simulink model "CCModel_71"  (R2024a)
settings: Solver=ode3  StartTime=0.0  StopTime=100  FixedStep=0.001  RelTol=1e-3  EnableMultiTasking=on
undefined symbols (not defined in the file or in its folder): DiscIntNeverNeededParam, Hecate_desVel1, Hecate_desVel2, Hecate_desVel3, Hecate_horShift, Hecate_period, Hecate_slope, Hecate_Transition1, Hecate_Transition2, Hecate_verShift, i, PME_qb, qb_map, RPM_qb, V
libraries: simulink x46
(part 6 of 11)

== system CCModel_71/Cruise Control/Version 7.3/PID Controller ==
  Error : Inport
  Source : Inport  Port=2
  Desired Velocity : Inport  Port=3
  Add : Sum
  Derivative : Derivative
  Gain : Gain  Gain=0.17
  Integrator : Integrator  ExternalReset=rising
  Kd : Gain  Gain=0.1
  Ki : Gain  Gain=0.0075
  Kp : Gain  Gain=4.2
  Polynomial : Polyval  Coefs=[0.0000428571, -0.0079428571, 0.5357142857, 0]
  Sum : Sum  Inputs=+++
  Switch : Switch  Criteria=u2 > Threshold  Threshold=100  SaturateOnIntegerOverflow=off  InputSameDT=off
  Throttle Adjustment : Subsystem
  u : Outport
  wires:
  Integrator/1 -> Ki/1
  Error/1 -> Kp/1, Derivative/1, Integrator/1
  Derivative/1 -> Kd/1
  Source/1 -> Integrator/2  "Integral reset"
  Desired Velocity/1 -> Polynomial/1, Switch/2, Gain/1
  Sum/1 -> Add/1
  Add/1 -> u/1
  Switch/1 -> Add/2
  Gain/1 -> Switch/3
  Polynomial/1 -> Switch/1
  Kd/1 -> Sum/1  "D"
  Kp/1 -> Sum/2  "P"
  Ki/1 -> Sum/3  "I"

== system CCModel_71/Cruise Control/Version 7.3/Sigmoid ==
  U1 : Inport
  U2 : Inport  Port=2
  Change_time : Inport  Port=3
  Abs : Abs  SaturateOnIntegerOverflow=off
  Abs2 : Abs  SaturateOnIntegerOverflow=off
  Add Constant : Bias  Bias=1  SaturateOnIntegerOverflow=off
  Add Constant2 : Bias  Bias=1  SaturateOnIntegerOverflow=off
  Add Constant3 : Bias  Bias=1  SaturateOnIntegerOverflow=off
  Add3 : Sum
  Add4 : Sum  Inputs=+-
  Add5 : Sum
  Clock1 : Clock
  Constant : Constant
  Constant3 : Constant
  Divide : Product  Inputs=/*
  Divide1 : Product  Inputs=**
  Divide4 : Product  Inputs=*/
  Divide5 : Product  Inputs=**
  Divide6 : Product  Inputs=**
  Divide8 : Product  Inputs=*/
  Gain : Gain  Gain=1/2
  Gain1 : Gain  Gain=2
  Gain2 : Gain  Gain=1000
  Gain3 : Gain  Gain=0.001
  Gain5 : Gain  Gain=1/2
  K : Constant  Value=4
  Power{,3..5} (4 alike) : Math  Operator=pow
  Reciprocal : Product  Inputs=/
  Reciprocal2 : Product  Inputs=/
  Round1 : Rounding  Operator=round
  Saturation : Saturate  UpperLimit=100  LowerLimit=-100
  Subtract : Sum  Inputs=+-
  Subtract1 : Sum  Inputs=+-
  Subtract2 : Sum  Inputs=+-
  Sum1 : Sum  Inputs=|-+
  h : Constant
  u_out : Outport
  wires:
  Add5/1 -> Saturation/1
  h/1 -> Divide8/1, Abs2/1, Subtract/2
  Add3/1 -> Divide6/2
  Add4/1 -> Divide5/1
  Constant3/1 -> Add4/1, Add3/2
  Power5/1 -> Divide4/2
  Reciprocal2/1 -> Power5/2
  K/1 -> Reciprocal2/1, Power4/2, Power/2, Reciprocal/1
  Gain5/1 -> Divide6/1
  Change_time/1 -> Sum1/1
  Abs/1 -> Power4/1
  Clock1/1 -> Sum1/2
  Gain3/1 -> Subtract/1
  U2/1 -> Gain5/1, Divide1/2
  Round1/1 -> Gain3/1
  Power4/1 -> Add Constant/1
  Gain2/1 -> Round1/1
  Add Constant/1 -> Power5/1
  Subtract/1 -> Divide4/1, Abs/1
  U1/1 -> Subtract2/1
  Divide6/1 -> Add5/1
  Sum1/1 -> Gain2/1
  Divide4/1 -> Add3/1, Add4/2
  Abs2/1 -> Power/1
  Power/1 -> Add Constant2/1
  Add Constant2/1 -> Power3/1
  Reciprocal/1 -> Power3/2
  Power3/1 -> Divide8/2
  Divide8/1 -> Add Constant3/1
  Add Constant3/1 -> Gain/1
  Constant/1 -> Subtract1/1
  Gain/1 -> Gain1/1, Subtract1/2  "P"
  Divide1/1 -> Subtract2/2
  Subtract2/1 -> Divide/2
  Gain1/1 -> Divide/1
  Divide/1 -> Divide5/2
  Divide5/1 -> Add5/2
  Saturation/1 -> u_out/1
  Subtract1/1 -> Divide1/1

== system CCModel_71/Cruise Control/Version 7.3/Switches ==
  U : Inport
  Throttle_In : Inport  Port=2
  Brake_In : Inport  Port=3
  Add Constant : Bias  Bias=6  SaturateOnIntegerOverflow=off
  Brake_Switch1 : Switch  Criteria=u2 > Threshold  Threshold=30  SaturateOnIntegerOverflow=off  InputSameDT=off
  Brake_Switch3 : Switch  Criteria=u2 > Threshold  Threshold=5  SaturateOnIntegerOverflow=off  InputSameDT=off
  Constant1 : Constant  Value=0
  Gain : Gain  Gain=-1
  Gain3 : Gain  Gain=0.15
  Max1 : MinMax  Function=max  Inputs=2
  Polynomial : Polyval  Coefs=[-0.01,0.2,0,0]
  Polynomial1 : Polyval  Coefs=[6.66666666666666666666666666666666666e-7,-9.33333333333333333333333333333333e-05,0.0105,-0.448,6]
  Saturation : Saturate  UpperLimit=100  LowerLimit=-100
  Switch : Switch  Criteria=u2 > Threshold  Threshold=10  SaturateOnIntegerOverflow=off  InputSameDT=off
  Switch1 : Switch  Criteria=u2 > Threshold  Threshold=-20  SaturateOnIntegerOverflow=off  InputSameDT=off
  Throttle_Switch1 : Switch  Criteria=u2 > Threshold  SaturateOnIntegerOverflow=off  InputSameDT=off
  Throttle_Switch3 : Switch  Criteria=u2 > Threshold  Threshold=5  SaturateOnIntegerOverflow=off  InputSameDT=off
  To Workspace : ToWorkspace  VariableName=throttleout  SampleTime=-1
      settings: Save2DSignal=2-D array (concatenate along first dimension)
  To Workspace1 : ToWorkspace  VariableName=brakeout  SampleTime=-1
      settings: Save2DSignal=2-D array (concatenate along first dimension)
  Throttle : Outport
  Brake : Outport  Port=2
  wires:
  Throttle_Switch1/1 -> Add Constant/1
  Brake_Switch3/1 -> To Workspace1/1, Brake/1
  Brake_In/1 -> Brake_Switch3/1, Max1/2
  Throttle_In/1 -> Throttle_Switch3/1, Max1/1
  Throttle_Switch3/1 -> Saturation/1
  Constant1/1 -> Throttle_Switch1/3, Brake_Switch1/1
  Switch/1 -> Throttle_Switch1/1
  Polynomial/1 -> Switch/3
  Max1/1 -> Brake_Switch3/2, Throttle_Switch3/2
  Add Constant/1 -> Throttle_Switch3/3
  Gain/1 -> Switch1/3
  Polynomial1/1 -> Switch1/1
  Switch1/1 -> Brake_Switch1/3
  Brake_Switch1/1 -> Gain3/1
  Gain3/1 -> Brake_Switch3/3
  Saturation/1 -> To Workspace/1, Throttle/1
  U/1 -> Switch1/2, Brake_Switch1/2, Throttle_Switch1/2, Gain/1, Switch/2, Switch/1, Polynomial/1, Polynomial1/1

== system CCModel_71/Powertrain/EM0/efficiency ==
  Motor speed [rpm] : Inport
  "Torque [Nm] " : Inport  Port=2
  Abs : Abs  SaturateOnIntegerOverflow=off
  Abs2 : Abs  SaturateOnIntegerOverflow=off
  Inverter efficiency : Gain  Gain=0.97
  Inverter efficiency1 : Gain  Gain=0.97
  Multiply : Gain  Gain=1/9.5488
  Product{,1..2,5} (4 alike) : Product
  Product3 : Product  Inputs=3
  Product4 : Product  Inputs=3
  RPM to rad/s : Gain  Gain=0.104719755
  RPM to rad/s1 : Gain  Gain=0.104719755
  Saturation : Saturate  UpperLimit=inf  LowerLimit=0
  Saturation1 : Saturate  UpperLimit=0  LowerLimit=-inf
  Saturation2 : Saturate  UpperLimit=inf  LowerLimit=0
  Saturation3 : Saturate  UpperLimit=inf  LowerLimit=0
  Sign : Signum  ZeroCross=off
  Subtract : Sum  Inputs=+-
  Subtract1 : Sum  Inputs=+-
  Switch : Switch  Criteria=u2 > Threshold  ZeroCross=off  SaturateOnIntegerOverflow=off  InputSameDT=off
  Terminator : Terminator
  Terminator1 : Terminator
  divider : Subsystem
  divider1 : Subsystem
  motor efficiency map : Lookup_n-D  BreakpointsForDimension1=|  BreakpointsForDimension2="[1\t440.500000000000\t881\t1321.50000000000\t1762\t2202.50000000000\t2643\t3083.50000000000\t3524\t3964.50000000000\t4405\t4845.50000000000\t5286\t5726.50000000000\t6167\t6607.50000000000\t7048\t7488.50000000000\t7929\t8369.50000000000\t8810]"  Table=|  InternalRulePriority=Speed  RndMeth=Simplest
      BreakpointsForDimension1=|
      | [1
      | 6
      | 12
      | 18
      | 36
      | 54
      | 72
      | 90
      | 108
      | 126
      | 144
      | 162
      | 180
      | 198
      | 216
      | 234
      | 252
      | 270
      | 288
      | 306
      | 324
      | 342
      | 360]
      Table=|
      | [0.100000000000000	0.100000000000000	0.420000000000000	0.440000000000000	0.450000000000000	0.460000000000000	0.470000000000000	0.480000000000000	0.490000000000000	0.500000000000000	0.510000000000000	0.520000000000000	0.530000000000000	0.540000000000000	0.550000000000000	0.560000000000000	0.580000000000000	0.560000000000000	0.550000000000000	0.540000000000000	0.500000000000000
      | 0.740000000000000	0.750000000000000	0.750000000000000	0.760000000000000	0.763000000000000	0.767000000000000	0.780000000000000	0.780000000000000	0.780000000000000	0.780000000000000	0.780000000000000	0.770000000000000	0.770000000000000	0.770000000000000	0.769000000000000	0.769000000000000	0.765000000000000	0.760000000000000	0.750000000000000	0.730000000000000	0.720000000000000
      | 0.780000000000000	0.790000000000000	0.800000000000000	0.850000000000000	0.880000000000000	0.890000000000000	0.895000000000000	0.900000000000000	0.910000000000000	0.910000000000000	0.910000000000000	0.915000000000000	0.915000000000000	0.918000000000000	0.917000000000000	0.916000000000000	0.910000000000000	0.910000000000000	0.894000000000000	0.870000000000000	0.850000000000000
      | 0.800000000000000	0.870000000000000	0.902500000000000	0.942500000000000	0.945000000000000	0.945000000000000	0.945000000000000	0.945000000000000	0.945000000000000	0.947500000000000	0.945000000000000	0.945000000000000	0.945000000000000	0.945000000000000	0.945000000000000	0.937500000000000	0.920000000000000	0.910000000000000	0.898000000000000	0.890000000000000	0.840000000000000
      | 0.800000000000000	0.880000000000000	0.902500000000000	0.947500000000000	0.953000000000000	0.955000000000000	0.957500000000000	0.957500000000000	0.956000000000000	0.960000000000000	0.960000000000000	0.960000000000000	0.960000000000000	0.957500000000000	0.957500000000000	0.955000000000000	0.950000000000000	0.945000000000000	0.940000000000000	0.920000000000000	0.890000000000000
      | 0.780000000000000	0.880000000000000	0.902500000000000	0.947500000000000	0.952500000000000	0.957500000000000	0.960000000000000	0.962000000000000	0.962500000000000	0.964000000000000	0.965000000000000	0.965000000000000	0.965000000000000	0.965000000000000	0.962500000000000	0.958000000000000	0.957000000000000	0.951000000000000	0.947500000000000	0.945000000000000	0.940000000000000
      | 0.740000000000000	0.880000000000000	0.902500000000000	0.942500000000000	0.952500000000000	0.955000000000000	0.962000000000000	0.964000000000000	0.966000000000000	0.967000000000000	0.968000000000000	0.970000000000000	0.967000000000000	0.966000000000000	0.964000000000000	0.962000000000000	0.960000000000000	0.956000000000000	0.953000000000000	0.948000000000000	0.945000000000000
      | 0.700000000000000	0.870000000000000	0.902500000000000	0.945000000000000	0.947500000000000	0.952500000000000	0.960000000000000	0.962500000000000	0.965000000000000	0.966000000000000	0.968000000000000	0.970000000000000	0.967500000000000	0.966500000000000	0.965000000000000	0.962500000000000	0.960000000000000	0.955000000000000	0.952000000000000	0.946000000000000	0.945000000000000
      | 0.650000000000000	0.860000000000000	0.902500000000000	0.932500000000000	0.942500000000000	0.950000000000000	0.957500000000000	0.961000000000000	0.963000000000000	0.965500000000000	0.967500000000000	0.970000000000000	0.967500000000000	0.965000000000000	0.964000000000000	0.960000000000000	0.957000000000000	0.953000000000000	0.950000000000000	0.945000000000000	0.942000000000000
      | 0.600000000000000	0.850000000000000	0.902500000000000	0.927500000000000	0.937500000000000	0.947500000000000	0.955000000000000	0.959000000000000	0.962500000000000	0.965000000000000	0.966000000000000	0.967500000000000	0.965000000000000	0.963000000000000	0.961800000000000	0.957500000000000	0.955000000000000	0.950000000000000	0.945000000000000	0.941000000000000	0.937500000000000
      | 0.590000000000000	0.840000000000000	0.902500000000000	0.925000000000000	0.932500000000000	0.942500000000000	0.952500000000000	0.957500000000000	0.960000000000000	0.962500000000000	0.965000000000000	0.965000000000000	0.962500000000000	0.961000000000000	0.958000000000000	0.954000000000000	0.950000000000000	0.945000000000000	0.940000000000000	0.930000000000000	0.925000000000000
      | 0.550000000000000	0.830000000000000	0.902500000000000	0.922500000000000	0.927500000000000	0.937500000000000	0.950000000000000	0.955000000000000	0.957500000000000	0.961000000000000	0.962500000000000	0.962500000000000	0.960000000000000	0.957500000000000	0.955000000000000	0.950000000000000	0.945000000000000	0.935000000000000	0.922500000000000	0.917500000000000	0.915000000000000
      | 0.540000000000000	0.820000000000000	0.890000000000000	0.920000000000000	0.922500000000000	0.935000000000000	0.947000000000000	0.952000000000000	0.955000000000000	0.958000000000000	0.961200000000000	0.960000000000000	0.957500000000000	0.954000000000000	0.950000000000000	0.942500000000000	0.932500000000000	0.922500000000000	0.912500000000000	0.910000000000000	0
      | 0.500000000000000	0.810000000000000	0.880000000000000	0.910000000000000	0.920000000000000	0.930000000000000	0.942500000000000	0.951250000000000	0.952500000000000	0.956000000000000	0.960000000000000	0.956000000000000	0.952500000000000	0.950000000000000	0.942500000000000	0.930000000000000	0.915000000000000	0.910000000000000	0	0	0
      | 0.450000000000000	0.805000000000000	0.870000000000000	0.905000000000000	0.917500000000000	0.925000000000000	0.940000000000000	0.945000000000000	0.950000000000000	0.952500000000000	0.955000000000000	0.952500000000000	0.948000000000000	0.942500000000000	0.930000000000000	0.915000000000000	0.910000000000000	0	0	0	0
      | 0.430000000000000	0.800000000000000	0.860000000000000	0.890000000000000	0.912500000000000	0.920000000000000	0.935000000000000	0.942500000000000	0.946000000000000	0.950000000000000	0.952500000000000	0.949000000000000	0.942500000000000	0.935000000000000	0.917500000000000	0.912500000000000	0	0	0	0	0
      | 0.420000000000000	0.790000000000000	0.850000000000000	0.880000000000000	0.907500000000000	0.915000000000000	0.932000000000000	0.937500000000000	0.942500000000000	0.945000000000000	0.948000000000000	0.942500000000000	0.935000000000000	0.922500000000000	0.915000000000000	0	0	0	0	0	0
      | 0.410000000000000	0.780000000000000	0.840000000000000	0.870000000000000	0.900000000000000	0.910000000000000	0.927500000000000	0.935000000000000	0.938000000000000	0.942500000000000	0.945000000000000	0.935000000000000	0.925000000000000	0.920000000000000	0	0	0	0	0	0	0
      | 0.400000000000000	0.760000000000000	0.830000000000000	0.860000000000000	0.890000000000000	0.905000000000000	0.922500000000000	0.930000000000000	0.935000000000000	0.937500000000000	0.935000000000000	0.927500000000000	0	0	0	0	0	0	0	0	0
      | 0.380000000000000	0.740000000000000	0.820000000000000	0.850000000000000	0.880000000000000	0.900000000000000	0.917500000000000	0.927500000000000	0.930000000000000	0.930000000000000	0.922500000000000	0.920000000000000	0	0	0	0	0	0	0	0	0
      | 0.360000000000000	0.710000000000000	0.810000000000000	0.840000000000000	0.875000000000000	0.897500000000000	0.912500000000000	0.922500000000000	0.925000000000000	0.928000000000000	0.915000000000000	0	0	0	0	0	0	0	0	0	0
      | 0.350000000000000	0.700000000000000	0.800000000000000	0.835000000000000	0.872500000000000	0.880000000000000	0.905000000000000	0.917500000000000	0.921000000000000	0.920000000000000	0	0	0	0	0	0	0	0	0	0	0
      | 0.350000000000000	0.680000000000000	0.790000000000000	0.830000000000000	0.870000000000000	0.875000000000000	0.900000000000000	0.910000000000000	0.900000000000000	0	0	0	0	0	0	0	0	0	0	0	0]
      settings: InputPortMap=u0,u1
  motor efficiency map1 : Lookup_n-D  BreakpointsForDimension1=|  BreakpointsForDimension2="[1\t440.500000000000\t881\t1321.50000000000\t1762\t2202.50000000000\t2643\t3083.50000000000\t3524\t3964.50000000000\t4405\t4845.50000000000\t5286\t5726.50000000000\t6167\t6607.50000000000\t7048\t7488.50000000000\t7929\t8369.50000000000\t8810]"  Table=|  InternalRulePriority=Speed  RndMeth=Simplest
      BreakpointsForDimension1=|
      | [1
      | 6
      | 12
      | 18
      | 36
      | 54
      | 72
      | 90
      | 108
      | 126
      | 144
      | 162
      | 180
      | 198
      | 216
      | 234
      | 252
      | 270
      | 288
      | 306
      | 324
      | 342
      | 360]
      Table=|
      | [0.100000000000000	0.100000000000000	0.420000000000000	0.440000000000000	0.450000000000000	0.460000000000000	0.470000000000000	0.480000000000000	0.490000000000000	0.500000000000000	0.510000000000000	0.520000000000000	0.530000000000000	0.540000000000000	0.550000000000000	0.560000000000000	0.580000000000000	0.560000000000000	0.550000000000000	0.540000000000000	0.500000000000000
      | 0.740000000000000	0.750000000000000	0.750000000000000	0.760000000000000	0.763000000000000	0.767000000000000	0.780000000000000	0.780000000000000	0.780000000000000	0.780000000000000	0.780000000000000	0.770000000000000	0.770000000000000	0.770000000000000	0.769000000000000	0.769000000000000	0.765000000000000	0.760000000000000	0.750000000000000	0.730000000000000	0.720000000000000
      | 0.780000000000000	0.790000000000000	0.800000000000000	0.850000000000000	0.880000000000000	0.890000000000000	0.895000000000000	0.900000000000000	0.910000000000000	0.910000000000000	0.910000000000000	0.915000000000000	0.915000000000000	0.918000000000000	0.917000000000000	0.916000000000000	0.910000000000000	0.910000000000000	0.894000000000000	0.870000000000000	0.850000000000000
      | 0.800000000000000	0.870000000000000	0.902500000000000	0.942500000000000	0.945000000000000	0.945000000000000	0.945000000000000	0.945000000000000	0.945000000000000	0.947500000000000	0.945000000000000	0.945000000000000	0.945000000000000	0.945000000000000	0.945000000000000	0.937500000000000	0.920000000000000	0.910000000000000	0.898000000000000	0.890000000000000	0.840000000000000
      | 0.800000000000000	0.880000000000000	0.902500000000000	0.947500000000000	0.953000000000000	0.955000000000000	0.957500000000000	0.957500000000000	0.956000000000000	0.960000000000000	0.960000000000000	0.960000000000000	0.960000000000000	0.957500000000000	0.957500000000000	0.955000000000000	0.950000000000000	0.945000000000000	0.940000000000000	0.920000000000000	0.890000000000000
      | 0.780000000000000	0.880000000000000	0.902500000000000	0.947500000000000	0.952500000000000	0.957500000000000	0.960000000000000	0.962000000000000	0.962500000000000	0.964000000000000	0.965000000000000	0.965000000000000	0.965000000000000	0.965000000000000	0.962500000000000	0.958000000000000	0.957000000000000	0.951000000000000	0.947500000000000	0.945000000000000	0.940000000000000
      | 0.740000000000000	0.880000000000000	0.902500000000000	0.942500000000000	0.952500000000000	0.955000000000000	0.962000000000000	0.964000000000000	0.966000000000000	0.967000000000000	0.968000000000000	0.970000000000000	0.967000000000000	0.966000000000000	0.964000000000000	0.962000000000000	0.960000000000000	0.956000000000000	0.953000000000000	0.948000000000000	0.945000000000000
      | 0.700000000000000	0.870000000000000	0.902500000000000	0.945000000000000	0.947500000000000	0.952500000000000	0.960000000000000	0.962500000000000	0.965000000000000	0.966000000000000	0.968000000000000	0.970000000000000	0.967500000000000	0.966500000000000	0.965000000000000	0.962500000000000	0.960000000000000	0.955000000000000	0.952000000000000	0.946000000000000	0.945000000000000
      | 0.650000000000000	0.860000000000000	0.902500000000000	0.932500000000000	0.942500000000000	0.950000000000000	0.957500000000000	0.961000000000000	0.963000000000000	0.965500000000000	0.967500000000000	0.970000000000000	0.967500000000000	0.965000000000000	0.964000000000000	0.960000000000000	0.957000000000000	0.953000000000000	0.950000000000000	0.945000000000000	0.942000000000000
      | 0.600000000000000	0.850000000000000	0.902500000000000	0.927500000000000	0.937500000000000	0.947500000000000	0.955000000000000	0.959000000000000	0.962500000000000	0.965000000000000	0.966000000000000	0.967500000000000	0.965000000000000	0.963000000000000	0.961800000000000	0.957500000000000	0.955000000000000	0.950000000000000	0.945000000000000	0.941000000000000	0.937500000000000
      | 0.590000000000000	0.840000000000000	0.902500000000000	0.925000000000000	0.932500000000000	0.942500000000000	0.952500000000000	0.957500000000000	0.960000000000000	0.962500000000000	0.965000000000000	0.965000000000000	0.962500000000000	0.961000000000000	0.958000000000000	0.954000000000000	0.950000000000000	0.945000000000000	0.940000000000000	0.930000000000000	0.925000000000000
      | 0.550000000000000	0.830000000000000	0.902500000000000	0.922500000000000	0.927500000000000	0.937500000000000	0.950000000000000	0.955000000000000	0.957500000000000	0.961000000000000	0.962500000000000	0.962500000000000	0.960000000000000	0.957500000000000	0.955000000000000	0.950000000000000	0.945000000000000	0.935000000000000	0.922500000000000	0.917500000000000	0.915000000000000
      | 0.540000000000000	0.820000000000000	0.890000000000000	0.920000000000000	0.922500000000000	0.935000000000000	0.947000000000000	0.952000000000000	0.955000000000000	0.958000000000000	0.961200000000000	0.960000000000000	0.957500000000000	0.954000000000000	0.950000000000000	0.942500000000000	0.932500000000000	0.922500000000000	0.912500000000000	0.910000000000000	0
      | 0.500000000000000	0.810000000000000	0.880000000000000	0.910000000000000	0.920000000000000	0.930000000000000	0.942500000000000	0.951250000000000	0.952500000000000	0.956000000000000	0.960000000000000	0.956000000000000	0.952500000000000	0.950000000000000	0.942500000000000	0.930000000000000	0.915000000000000	0.910000000000000	0	0	0
      | 0.450000000000000	0.805000000000000	0.870000000000000	0.905000000000000	0.917500000000000	0.925000000000000	0.940000000000000	0.945000000000000	0.950000000000000	0.952500000000000	0.955000000000000	0.952500000000000	0.948000000000000	0.942500000000000	0.930000000000000	0.915000000000000	0.910000000000000	0	0	0	0
      | 0.430000000000000	0.800000000000000	0.860000000000000	0.890000000000000	0.912500000000000	0.920000000000000	0.935000000000000	0.942500000000000	0.946000000000000	0.950000000000000	0.952500000000000	0.949000000000000	0.942500000000000	0.935000000000000	0.917500000000000	0.912500000000000	0	0	0	0	0
      | 0.420000000000000	0.790000000000000	0.850000000000000	0.880000000000000	0.907500000000000	0.915000000000000	0.932000000000000	0.937500000000000	0.942500000000000	0.945000000000000	0.948000000000000	0.942500000000000	0.935000000000000	0.922500000000000	0.915000000000000	0	0	0	0	0	0
      | 0.410000000000000	0.780000000000000	0.840000000000000	0.870000000000000	0.900000000000000	0.910000000000000	0.927500000000000	0.935000000000000	0.938000000000000	0.942500000000000	0.945000000000000	0.935000000000000	0.925000000000000	0.920000000000000	0	0	0	0	0	0	0
      | 0.400000000000000	0.760000000000000	0.830000000000000	0.860000000000000	0.890000000000000	0.905000000000000	0.922500000000000	0.930000000000000	0.935000000000000	0.937500000000000	0.935000000000000	0.927500000000000	0	0	0	0	0	0	0	0	0
      | 0.380000000000000	0.740000000000000	0.820000000000000	0.850000000000000	0.880000000000000	0.900000000000000	0.917500000000000	0.927500000000000	0.930000000000000	0.930000000000000	0.922500000000000	0.920000000000000	0	0	0	0	0	0	0	0	0
      | 0.360000000000000	0.710000000000000	0.810000000000000	0.840000000000000	0.875000000000000	0.897500000000000	0.912500000000000	0.922500000000000	0.925000000000000	0.928000000000000	0.915000000000000	0	0	0	0	0	0	0	0	0	0
      | 0.350000000000000	0.700000000000000	0.800000000000000	0.835000000000000	0.872500000000000	0.880000000000000	0.905000000000000	0.917500000000000	0.921000000000000	0.920000000000000	0	0	0	0	0	0	0	0	0	0	0
      | 0.350000000000000	0.680000000000000	0.790000000000000	0.830000000000000	0.870000000000000	0.875000000000000	0.900000000000000	0.910000000000000	0.900000000000000	0	0	0	0	0	0	0	0	0	0	0	0]
      settings: InputPortMap=u0,u1
  Electrical power [W] : Outport
  wires:
  Switch/1 -> Electrical power [W]/1  "Elec_power"
  Sign/1 -> Switch/2
  Product1/1 -> Switch/3
  divider/1(Out1) -> Switch/1
  "Torque [Nm] "/1 -> Abs/1, Product5/1, Product4/2, Abs2/1, Product3/1, Product2/2, Product/2
  Product/1 -> Multiply/1
  motor efficiency map/1 -> Saturation2/1
  motor efficiency map1/1 -> Saturation3/1
  Abs/1 -> motor efficiency map1/1
  Motor speed [rpm]/1 -> motor efficiency map1/2, RPM to rad/s1/1, Product/1, RPM to rad/s/1, motor efficiency map/2
  Saturation3/1 -> Inverter efficiency1/1
  Saturation2/1 -> Inverter efficiency/1
  Abs2/1 -> motor efficiency map/1
  RPM to rad/s/1 -> Product3/2, Product2/1
  Product3/1 -> Subtract/2
  Product2/1 -> Subtract/1
  Subtract/1 -> divider1/1(In1)
  divider1/1(Out1) -> Saturation/1  "propelling"
  RPM to rad/s1/1 -> Product5/2, Product4/3
  Product4/1 -> Subtract1/1
  Product5/1 -> Subtract1/2
  Subtract1/1 -> Saturation1/1  "ReGen"
  Multiply/1 -> Product1/1, Sign/1, divider/1(In1)  "Mech_power"
  Inverter efficiency/1 -> divider1/2(In2), Product3/3, divider/2(In2)
  Inverter efficiency1/1 -> Product4/1, Product1/2
  Saturation/1 -> Terminator/1
  Saturation1/1 -> Terminator1/1

== system CCModel_71/Powertrain/EM1/efficiency ==
  Motor speed [rpm] : Inport
  "Torque [Nm] " : Inport  Port=2
  Abs : Abs  SaturateOnIntegerOverflow=off
  Abs2 : Abs  SaturateOnIntegerOverflow=off
  Inverter efficiency : Gain  Gain=0.97
  Inverter efficiency1 : Gain  Gain=0.97
  Multiply : Gain  Gain=1/9.5488
  Product{,1..2,5} (4 alike) : Product
  Product3 : Product  Inputs=3
  Product4 : Product  Inputs=3
  RPM to rad/s : Gain  Gain=0.104719755
  RPM to rad/s1 : Gain  Gain=0.104719755
  Saturation : Saturate  UpperLimit=inf  LowerLimit=0
  Saturation1 : Saturate  UpperLimit=0  LowerLimit=-inf
  Saturation2 : Saturate  UpperLimit=inf  LowerLimit=0
  Saturation3 : Saturate  UpperLimit=inf  LowerLimit=0
  Sign : Signum  ZeroCross=off
  Subtract : Sum  Inputs=+-
  Subtract1 : Sum  Inputs=+-
  Switch : Switch  Criteria=u2 > Threshold  ZeroCross=off  SaturateOnIntegerOverflow=off  InputSameDT=off
  Terminator : Terminator
  Terminator1 : Terminator
  divider : Subsystem
  divider1 : Subsystem
  motor efficiency map : Lookup_n-D  BreakpointsForDimension1=|  BreakpointsForDimension2="[1\t440.500000000000\t881\t1321.50000000000\t1762\t2202.50000000000\t2643\t3083.50000000000\t3524\t3964.50000000000\t4405\t4845.50000000000\t5286\t5726.50000000000\t6167\t6607.50000000000\t7048\t7488.50000000000\t7929\t8369.50000000000\t8810]"  Table=|  InternalRulePriority=Speed  RndMeth=Simplest
      BreakpointsForDimension1=|
      | [1
      | 6
      | 12
      | 18
      | 36
      | 54
      | 72
      | 90
      | 108
      | 126
      | 144
      | 162
      | 180
      | 198
      | 216
      | 234
      | 252
      | 270
      | 288
      | 306
      | 324
      | 342
      | 360]
      Table=|
      | [0.100000000000000	0.100000000000000	0.420000000000000	0.440000000000000	0.450000000000000	0.460000000000000	0.470000000000000	0.480000000000000	0.490000000000000	0.500000000000000	0.510000000000000	0.520000000000000	0.530000000000000	0.540000000000000	0.550000000000000	0.560000000000000	0.580000000000000	0.560000000000000	0.550000000000000	0.540000000000000	0.500000000000000
      | 0.740000000000000	0.750000000000000	0.750000000000000	0.760000000000000	0.763000000000000	0.767000000000000	0.780000000000000	0.780000000000000	0.780000000000000	0.780000000000000	0.780000000000000	0.770000000000000	0.770000000000000	0.770000000000000	0.769000000000000	0.769000000000000	0.765000000000000	0.760000000000000	0.750000000000000	0.730000000000000	0.720000000000000
      | 0.780000000000000	0.790000000000000	0.800000000000000	0.850000000000000	0.880000000000000	0.890000000000000	0.895000000000000	0.900000000000000	0.910000000000000	0.910000000000000	0.910000000000000	0.915000000000000	0.915000000000000	0.918000000000000	0.917000000000000	0.916000000000000	0.910000000000000	0.910000000000000	0.894000000000000	0.870000000000000	0.850000000000000
      | 0.800000000000000	0.870000000000000	0.902500000000000	0.942500000000000	0.945000000000000	0.945000000000000	0.945000000000000	0.945000000000000	0.945000000000000	0.947500000000000	0.945000000000000	0.945000000000000	0.945000000000000	0.945000000000000	0.945000000000000	0.937500000000000	0.920000000000000	0.910000000000000	0.898000000000000	0.890000000000000	0.840000000000000
      | 0.800000000000000	0.880000000000000	0.902500000000000	0.947500000000000	0.953000000000000	0.955000000000000	0.957500000000000	0.957500000000000	0.956000000000000	0.960000000000000	0.960000000000000	0.960000000000000	0.960000000000000	0.957500000000000	0.957500000000000	0.955000000000000	0.950000000000000	0.945000000000000	0.940000000000000	0.920000000000000	0.890000000000000
      | 0.780000000000000	0.880000000000000	0.902500000000000	0.947500000000000	0.952500000000000	0.957500000000000	0.960000000000000	0.962000000000000	0.962500000000000	0.964000000000000	0.965000000000000	0.965000000000000	0.965000000000000	0.965000000000000	0.962500000000000	0.958000000000000	0.957000000000000	0.951000000000000	0.947500000000000	0.945000000000000	0.940000000000000
      | 0.740000000000000	0.880000000000000	0.902500000000000	0.942500000000000	0.952500000000000	0.955000000000000	0.962000000000000	0.964000000000000	0.966000000000000	0.967000000000000	0.968000000000000	0.970000000000000	0.967000000000000	0.966000000000000	0.964000000000000	0.962000000000000	0.960000000000000	0.956000000000000	0.953000000000000	0.948000000000000	0.945000000000000
      | 0.700000000000000	0.870000000000000	0.902500000000000	0.945000000000000	0.947500000000000	0.952500000000000	0.960000000000000	0.962500000000000	0.965000000000000	0.966000000000000	0.968000000000000	0.970000000000000	0.967500000000000	0.966500000000000	0.965000000000000	0.962500000000000	0.960000000000000	0.955000000000000	0.952000000000000	0.946000000000000	0.945000000000000
      | 0.650000000000000	0.860000000000000	0.902500000000000	0.932500000000000	0.942500000000000	0.950000000000000	0.957500000000000	0.961000000000000	0.963000000000000	0.965500000000000	0.967500000000000	0.970000000000000	0.967500000000000	0.965000000000000	0.964000000000000	0.960000000000000	0.957000000000000	0.953000000000000	0.950000000000000	0.945000000000000	0.942000000000000
      | 0.600000000000000	0.850000000000000	0.902500000000000	0.927500000000000	0.937500000000000	0.947500000000000	0.955000000000000	0.959000000000000	0.962500000000000	0.965000000000000	0.966000000000000	0.967500000000000	0.965000000000000	0.963000000000000	0.961800000000000	0.957500000000000	0.955000000000000	0.950000000000000	0.945000000000000	0.941000000000000	0.937500000000000
      | 0.590000000000000	0.840000000000000	0.902500000000000	0.925000000000000	0.932500000000000	0.942500000000000	0.952500000000000	0.957500000000000	0.960000000000000	0.962500000000000	0.965000000000000	0.965000000000000	0.962500000000000	0.961000000000000	0.958000000000000	0.954000000000000	0.950000000000000	0.945000000000000	0.940000000000000	0.930000000000000	0.925000000000000
      | 0.550000000000000	0.830000000000000	0.902500000000000	0.922500000000000	0.927500000000000	0.937500000000000	0.950000000000000	0.955000000000000	0.957500000000000	0.961000000000000	0.962500000000000	0.962500000000000	0.960000000000000	0.957500000000000	0.955000000000000	0.950000000000000	0.945000000000000	0.935000000000000	0.922500000000000	0.917500000000000	0.915000000000000
      | 0.540000000000000	0.820000000000000	0.890000000000000	0.920000000000000	0.922500000000000	0.935000000000000	0.947000000000000	0.952000000000000	0.955000000000000	0.958000000000000	0.961200000000000	0.960000000000000	0.957500000000000	0.954000000000000	0.950000000000000	0.942500000000000	0.932500000000000	0.922500000000000	0.912500000000000	0.910000000000000	0
      | 0.500000000000000	0.810000000000000	0.880000000000000	0.910000000000000	0.920000000000000	0.930000000000000	0.942500000000000	0.951250000000000	0.952500000000000	0.956000000000000	0.960000000000000	0.956000000000000	0.952500000000000	0.950000000000000	0.942500000000000	0.930000000000000	0.915000000000000	0.910000000000000	0	0	0
      | 0.450000000000000	0.805000000000000	0.870000000000000	0.905000000000000	0.917500000000000	0.925000000000000	0.940000000000000	0.945000000000000	0.950000000000000	0.952500000000000	0.955000000000000	0.952500000000000	0.948000000000000	0.942500000000000	0.930000000000000	0.915000000000000	0.910000000000000	0	0	0	0
      | 0.430000000000000	0.800000000000000	0.860000000000000	0.890000000000000	0.912500000000000	0.920000000000000	0.935000000000000	0.942500000000000	0.946000000000000	0.950000000000000	0.952500000000000	0.949000000000000	0.942500000000000	0.935000000000000	0.917500000000000	0.912500000000000	0	0	0	0	0
      | 0.420000000000000	0.790000000000000	0.850000000000000	0.880000000000000	0.907500000000000	0.915000000000000	0.932000000000000	0.937500000000000	0.942500000000000	0.945000000000000	0.948000000000000	0.942500000000000	0.935000000000000	0.922500000000000	0.915000000000000	0	0	0	0	0	0
      | 0.410000000000000	0.780000000000000	0.840000000000000	0.870000000000000	0.900000000000000	0.910000000000000	0.927500000000000	0.935000000000000	0.938000000000000	0.942500000000000	0.945000000000000	0.935000000000000	0.925000000000000	0.920000000000000	0	0	0	0	0	0	0
      | 0.400000000000000	0.760000000000000	0.830000000000000	0.860000000000000	0.890000000000000	0.905000000000000	0.922500000000000	0.930000000000000	0.935000000000000	0.937500000000000	0.935000000000000	0.927500000000000	0	0	0	0	0	0	0	0	0
      | 0.380000000000000	0.740000000000000	0.820000000000000	0.850000000000000	0.880000000000000	0.900000000000000	0.917500000000000	0.927500000000000	0.930000000000000	0.930000000000000	0.922500000000000	0.920000000000000	0	0	0	0	0	0	0	0	0
      | 0.360000000000000	0.710000000000000	0.810000000000000	0.840000000000000	0.875000000000000	0.897500000000000	0.912500000000000	0.922500000000000	0.925000000000000	0.928000000000000	0.915000000000000	0	0	0	0	0	0	0	0	0	0
      | 0.350000000000000	0.700000000000000	0.800000000000000	0.835000000000000	0.872500000000000	0.880000000000000	0.905000000000000	0.917500000000000	0.921000000000000	0.920000000000000	0	0	0	0	0	0	0	0	0	0	0
      | 0.350000000000000	0.680000000000000	0.790000000000000	0.830000000000000	0.870000000000000	0.875000000000000	0.900000000000000	0.910000000000000	0.900000000000000	0	0	0	0	0	0	0	0	0	0	0	0]
      settings: InputPortMap=u0,u1
  motor efficiency map1 : Lookup_n-D  BreakpointsForDimension1=|  BreakpointsForDimension2="[1\t440.500000000000\t881\t1321.50000000000\t1762\t2202.50000000000\t2643\t3083.50000000000\t3524\t3964.50000000000\t4405\t4845.50000000000\t5286\t5726.50000000000\t6167\t6607.50000000000\t7048\t7488.50000000000\t7929\t8369.50000000000\t8810]"  Table=|  InternalRulePriority=Speed  RndMeth=Simplest
      BreakpointsForDimension1=|
      | [1
      | 6
      | 12
      | 18
      | 36
      | 54
      | 72
      | 90
      | 108
      | 126
      | 144
      | 162
      | 180
      | 198
      | 216
      | 234
      | 252
      | 270
      | 288
      | 306
      | 324
      | 342
      | 360]
      Table=|
      | [0.100000000000000	0.100000000000000	0.420000000000000	0.440000000000000	0.450000000000000	0.460000000000000	0.470000000000000	0.480000000000000	0.490000000000000	0.500000000000000	0.510000000000000	0.520000000000000	0.530000000000000	0.540000000000000	0.550000000000000	0.560000000000000	0.580000000000000	0.560000000000000	0.550000000000000	0.540000000000000	0.500000000000000
      | 0.740000000000000	0.750000000000000	0.750000000000000	0.760000000000000	0.763000000000000	0.767000000000000	0.780000000000000	0.780000000000000	0.780000000000000	0.780000000000000	0.780000000000000	0.770000000000000	0.770000000000000	0.770000000000000	0.769000000000000	0.769000000000000	0.765000000000000	0.760000000000000	0.750000000000000	0.730000000000000	0.720000000000000
      | 0.780000000000000	0.790000000000000	0.800000000000000	0.850000000000000	0.880000000000000	0.890000000000000	0.895000000000000	0.900000000000000	0.910000000000000	0.910000000000000	0.910000000000000	0.915000000000000	0.915000000000000	0.918000000000000	0.917000000000000	0.916000000000000	0.910000000000000	0.910000000000000	0.894000000000000	0.870000000000000	0.850000000000000
      | 0.800000000000000	0.870000000000000	0.902500000000000	0.942500000000000	0.945000000000000	0.945000000000000	0.945000000000000	0.945000000000000	0.945000000000000	0.947500000000000	0.945000000000000	0.945000000000000	0.945000000000000	0.945000000000000	0.945000000000000	0.937500000000000	0.920000000000000	0.910000000000000	0.898000000000000	0.890000000000000	0.840000000000000
      | 0.800000000000000	0.880000000000000	0.902500000000000	0.947500000000000	0.953000000000000	0.955000000000000	0.957500000000000	0.957500000000000	0.956000000000000	0.960000000000000	0.960000000000000	0.960000000000000	0.960000000000000	0.957500000000000	0.957500000000000	0.955000000000000	0.950000000000000	0.945000000000000	0.940000000000000	0.920000000000000	0.890000000000000
      | 0.780000000000000	0.880000000000000	0.902500000000000	0.947500000000000	0.952500000000000	0.957500000000000	0.960000000000000	0.962000000000000	0.962500000000000	0.964000000000000	0.965000000000000	0.965000000000000	0.965000000000000	0.965000000000000	0.962500000000000	0.958000000000000	0.957000000000000	0.951000000000000	0.947500000000000	0.945000000000000	0.940000000000000
      | 0.740000000000000	0.880000000000000	0.902500000000000	0.942500000000000	0.952500000000000	0.955000000000000	0.962000000000000	0.964000000000000	0.966000000000000	0.967000000000000	0.968000000000000	0.970000000000000	0.967000000000000	0.966000000000000	0.964000000000000	0.962000000000000	0.960000000000000	0.956000000000000	0.953000000000000	0.948000000000000	0.945000000000000
      | 0.700000000000000	0.870000000000000	0.902500000000000	0.945000000000000	0.947500000000000	0.952500000000000	0.960000000000000	0.962500000000000	0.965000000000000	0.966000000000000	0.968000000000000	0.970000000000000	0.967500000000000	0.966500000000000	0.965000000000000	0.962500000000000	0.960000000000000	0.955000000000000	0.952000000000000	0.946000000000000	0.945000000000000
      | 0.650000000000000	0.860000000000000	0.902500000000000	0.932500000000000	0.942500000000000	0.950000000000000	0.957500000000000	0.961000000000000	0.963000000000000	0.965500000000000	0.967500000000000	0.970000000000000	0.967500000000000	0.965000000000000	0.964000000000000	0.960000000000000	0.957000000000000	0.953000000000000	0.950000000000000	0.945000000000000	0.942000000000000
      | 0.600000000000000	0.850000000000000	0.902500000000000	0.927500000000000	0.937500000000000	0.947500000000000	0.955000000000000	0.959000000000000	0.962500000000000	0.965000000000000	0.966000000000000	0.967500000000000	0.965000000000000	0.963000000000000	0.961800000000000	0.957500000000000	0.955000000000000	0.950000000000000	0.945000000000000	0.941000000000000	0.937500000000000
      | 0.590000000000000	0.840000000000000	0.902500000000000	0.925000000000000	0.932500000000000	0.942500000000000	0.952500000000000	0.957500000000000	0.960000000000000	0.962500000000000	0.965000000000000	0.965000000000000	0.962500000000000	0.961000000000000	0.958000000000000	0.954000000000000	0.950000000000000	0.945000000000000	0.940000000000000	0.930000000000000	0.925000000000000
      | 0.550000000000000	0.830000000000000	0.902500000000000	0.922500000000000	0.927500000000000	0.937500000000000	0.950000000000000	0.955000000000000	0.957500000000000	0.961000000000000	0.962500000000000	0.962500000000000	0.960000000000000	0.957500000000000	0.955000000000000	0.950000000000000	0.945000000000000	0.935000000000000	0.922500000000000	0.917500000000000	0.915000000000000
      | 0.540000000000000	0.820000000000000	0.890000000000000	0.920000000000000	0.922500000000000	0.935000000000000	0.947000000000000	0.952000000000000	0.955000000000000	0.958000000000000	0.961200000000000	0.960000000000000	0.957500000000000	0.954000000000000	0.950000000000000	0.942500000000000	0.932500000000000	0.922500000000000	0.912500000000000	0.910000000000000	0
      | 0.500000000000000	0.810000000000000	0.880000000000000	0.910000000000000	0.920000000000000	0.930000000000000	0.942500000000000	0.951250000000000	0.952500000000000	0.956000000000000	0.960000000000000	0.956000000000000	0.952500000000000	0.950000000000000	0.942500000000000	0.930000000000000	0.915000000000000	0.910000000000000	0	0	0
      | 0.450000000000000	0.805000000000000	0.870000000000000	0.905000000000000	0.917500000000000	0.925000000000000	0.940000000000000	0.945000000000000	0.950000000000000	0.952500000000000	0.955000000000000	0.952500000000000	0.948000000000000	0.942500000000000	0.930000000000000	0.915000000000000	0.910000000000000	0	0	0	0
      | 0.430000000000000	0.800000000000000	0.860000000000000	0.890000000000000	0.912500000000000	0.920000000000000	0.935000000000000	0.942500000000000	0.946000000000000	0.950000000000000	0.952500000000000	0.949000000000000	0.942500000000000	0.935000000000000	0.917500000000000	0.912500000000000	0	0	0	0	0
      | 0.420000000000000	0.790000000000000	0.850000000000000	0.880000000000000	0.907500000000000	0.915000000000000	0.932000000000000	0.937500000000000	0.942500000000000	0.945000000000000	0.948000000000000	0.942500000000000	0.935000000000000	0.922500000000000	0.915000000000000	0	0	0	0	0	0
      | 0.410000000000000	0.780000000000000	0.840000000000000	0.870000000000000	0.900000000000000	0.910000000000000	0.927500000000000	0.935000000000000	0.938000000000000	0.942500000000000	0.945000000000000	0.935000000000000	0.925000000000000	0.920000000000000	0	0	0	0	0	0	0
      | 0.400000000000000	0.760000000000000	0.830000000000000	0.860000000000000	0.890000000000000	0.905000000000000	0.922500000000000	0.930000000000000	0.935000000000000	0.937500000000000	0.935000000000000	0.927500000000000	0	0	0	0	0	0	0	0	0
      | 0.380000000000000	0.740000000000000	0.820000000000000	0.850000000000000	0.880000000000000	0.900000000000000	0.917500000000000	0.927500000000000	0.930000000000000	0.930000000000000	0.922500000000000	0.920000000000000	0	0	0	0	0	0	0	0	0
      | 0.360000000000000	0.710000000000000	0.810000000000000	0.840000000000000	0.875000000000000	0.897500000000000	0.912500000000000	0.922500000000000	0.925000000000000	0.928000000000000	0.915000000000000	0	0	0	0	0	0	0	0	0	0
      | 0.350000000000000	0.700000000000000	0.800000000000000	0.835000000000000	0.872500000000000	0.880000000000000	0.905000000000000	0.917500000000000	0.921000000000000	0.920000000000000	0	0	0	0	0	0	0	0	0	0	0
      | 0.350000000000000	0.680000000000000	0.790000000000000	0.830000000000000	0.870000000000000	0.875000000000000	0.900000000000000	0.910000000000000	0.900000000000000	0	0	0	0	0	0	0	0	0	0	0	0]
      settings: InputPortMap=u0,u1
  Electrical power [W] : Outport
  wires:
  Switch/1 -> Electrical power [W]/1  "Elec_power"
  Sign/1 -> Switch/2
  Product1/1 -> Switch/3
  divider/1(Out1) -> Switch/1
  "Torque [Nm] "/1 -> Abs/1, Product5/1, Product4/2, Abs2/1, Product3/1, Product2/2, Product/2
  Product/1 -> Multiply/1
  motor efficiency map/1 -> Saturation2/1
  motor efficiency map1/1 -> Saturation3/1
  Abs/1 -> motor efficiency map1/1
  Motor speed [rpm]/1 -> motor efficiency map1/2, RPM to rad/s1/1, Product/1, RPM to rad/s/1, motor efficiency map/2
  Saturation3/1 -> Inverter efficiency1/1
  Saturation2/1 -> Inverter efficiency/1
  Abs2/1 -> motor efficiency map/1
  RPM to rad/s/1 -> Product3/2, Product2/1
  Product3/1 -> Subtract/2
  Product2/1 -> Subtract/1
  Subtract/1 -> divider1/1(In1)
  divider1/1(Out1) -> Saturation/1  "propelling"
  RPM to rad/s1/1 -> Product5/2, Product4/3
  Product4/1 -> Subtract1/1
  Product5/1 -> Subtract1/2
  Subtract1/1 -> Saturation1/1  "ReGen"
  Multiply/1 -> Product1/1, Sign/1, divider/1(In1)  "Mech_power"
  Inverter efficiency/1 -> divider1/2(In2), Product3/3, divider/2(In2)
  Inverter efficiency1/1 -> Product4/1, Product1/2
  Saturation/1 -> Terminator/1
  Saturation1/1 -> Terminator1/1
